simulink model "model"  (R2024b)
settings: Solver=ode1  StartTime=0.0  StopTime=10  FixedStep=0.0001  RelTol=1e-3
values from neighbouring files (symbols this model uses):
  a1 = c*a2    (= 810)    [init.m]
  a2 = c*a3    (= 270)    [init.m]
  a3 = c*a4    (= 90)    [init.m]
  a4 = c*10    (= 30)    [init.m]
  c1 = 50    [init.m]
  c2 = 1    [init.m]
  d = 100    [init.m]
  dis_gain = 30    [init.m]
  epsilon = 1    [init.m]
  i = 20    [init.m]
  k = 5    [init.m]
  mu = 0.9    [init.m]
  p = 400    [init.m]
  phi_frist = 0    [init.m]
  psi_frist = 0    [init.m]
  tau_p_max = 3000000    [init.m]
  theta_frist = 0    [init.m]
  umax = pi/2 - 0.01    (= 1.56079632679)    [init.m]
  w = wo    (= 50)    [init.m]
  wo = 50    [init.m]
  x_frist = 0    [init.m]
  y_frist = 0    [init.m]
  z_frist = 0    [init.m]
libraries: fod x36, slpidlib x6, simulink x1
(part 2 of 4)

== system model/FO_SMC/Subsystem/Subsystem1 ==
  y : Inport
  Constant : Constant  Value=a1
  Constant1 : Constant  Value=a2
  Constant2 : Constant  Value=a3
  Constant3 : Constant  Value=a4
  Demux : Demux
  Integrator : Integrator  InitialCondition=[0]
  MATLAB Function : MATLAB Function  TreatAsAtomicUnit=on
  Mux : Mux
  y_hat : Outport
  y1_hat : Outport  Port=2
  y1_hat1 : Outport  Port=3
  wires:
  Constant3/1 -> MATLAB Function/9(a4)
  Constant2/1 -> MATLAB Function/8(a3)
  Constant1/1 -> MATLAB Function/7(a2)
  Constant/1 -> MATLAB Function/6(a1)
  Demux/4 -> MATLAB Function/5(z4)
  MATLAB Function/4(z4_1) -> Mux/4
  Demux/3 -> MATLAB Function/4(z3), y1_hat1/1
  Integrator/1 -> Demux/1
  MATLAB Function/3(z3_1) -> Mux/3
  Demux/1 -> MATLAB Function/2(z1), y_hat/1
  MATLAB Function/1(z1_1) -> Mux/1
  MATLAB Function/2(z2_1) -> Mux/2
  Mux/1 -> Integrator/1
  Demux/2 -> MATLAB Function/3(z2), y1_hat/1
  y/1 -> MATLAB Function/1(x)

== system model/FO_SMC/Subsystem/Subsystem2 ==
  y : Inport
  Constant : Constant  Value=a1
  Constant1 : Constant  Value=a2
  Constant2 : Constant  Value=a3
  Constant3 : Constant  Value=a4
  Demux : Demux
  Integrator : Integrator  InitialCondition=[0]
  MATLAB Function : MATLAB Function  TreatAsAtomicUnit=on
  Mux : Mux
  y_hat : Outport
  y1_hat : Outport  Port=2
  y1_hat1 : Outport  Port=3
  wires:
  y/1 -> MATLAB Function/1(x)
  Demux/2 -> y1_hat/1, MATLAB Function/3(z2)
  Mux/1 -> Integrator/1
  MATLAB Function/2(z2_1) -> Mux/2
  MATLAB Function/1(z1_1) -> Mux/1
  Demux/1 -> y_hat/1, MATLAB Function/2(z1)
  MATLAB Function/3(z3_1) -> Mux/3
  Integrator/1 -> Demux/1
  Demux/3 -> y1_hat1/1, MATLAB Function/4(z3)
  MATLAB Function/4(z4_1) -> Mux/4
  Demux/4 -> MATLAB Function/5(z4)
  Constant/1 -> MATLAB Function/6(a1)
  Constant1/1 -> MATLAB Function/7(a2)
  Constant2/1 -> MATLAB Function/8(a3)
  Constant3/1 -> MATLAB Function/9(a4)

== system model/FO_SMC/Subsystem/Subsystem3 ==
  y : Inport
  Constant : Constant  Value=a1
  Constant1 : Constant  Value=a2
  Constant2 : Constant  Value=a3
  Constant3 : Constant  Value=a4
  Demux : Demux
  Integrator : Integrator  InitialCondition=[0]
  MATLAB Function : MATLAB Function  TreatAsAtomicUnit=on
  Mux : Mux
  y_hat : Outport
  y1_hat : Outport  Port=2
  y1_hat1 : Outport  Port=3
  wires:
  Constant3/1 -> MATLAB Function/9(a4)
  Constant2/1 -> MATLAB Function/8(a3)
  Constant1/1 -> MATLAB Function/7(a2)
  Constant/1 -> MATLAB Function/6(a1)
  Demux/4 -> MATLAB Function/5(z4)
  MATLAB Function/4(z4_1) -> Mux/4
  Demux/3 -> MATLAB Function/4(z3), y1_hat1/1
  Integrator/1 -> Demux/1
  MATLAB Function/3(z3_1) -> Mux/3
  Demux/1 -> MATLAB Function/2(z1), y_hat/1
  MATLAB Function/1(z1_1) -> Mux/1
  MATLAB Function/2(z2_1) -> Mux/2
  Mux/1 -> Integrator/1
  Demux/2 -> MATLAB Function/3(z2), y1_hat/1
  y/1 -> MATLAB Function/1(x)

== system model/FO_SMC/Subsystem/Subsystem4 ==
  y : Inport
  Constant : Constant  Value=a1
  Constant1 : Constant  Value=a2
  Constant2 : Constant  Value=a3
  Constant3 : Constant  Value=a4
  Demux : Demux
  Integrator : Integrator  InitialCondition=[0]
  MATLAB Function : MATLAB Function  TreatAsAtomicUnit=on
  Mux : Mux
  y_hat : Outport
  y1_hat : Outport  Port=2
  y1_hat1 : Outport  Port=3
  wires:
  y/1 -> MATLAB Function/1(x)
  Demux/2 -> y1_hat/1, MATLAB Function/3(z2)
  Mux/1 -> Integrator/1
  MATLAB Function/2(z2_1) -> Mux/2
  MATLAB Function/1(z1_1) -> Mux/1
  Demux/1 -> y_hat/1, MATLAB Function/2(z1)
  MATLAB Function/3(z3_1) -> Mux/3
  Integrator/1 -> Demux/1
  Demux/3 -> y1_hat1/1, MATLAB Function/4(z3)
  MATLAB Function/4(z4_1) -> Mux/4
  Demux/4 -> MATLAB Function/5(z4)
  Constant/1 -> MATLAB Function/6(a1)
  Constant1/1 -> MATLAB Function/7(a2)
  Constant2/1 -> MATLAB Function/8(a3)
  Constant3/1 -> MATLAB Function/9(a4)

== system model/FO_SMC/Subsystem/Subsystem5 ==
  y : Inport
  Constant : Constant  Value=a1
  Constant1 : Constant  Value=a2
  Constant2 : Constant  Value=a3
  Constant3 : Constant  Value=a4
  Demux : Demux
  Integrator : Integrator  InitialCondition=[0]
  MATLAB Function : MATLAB Function  TreatAsAtomicUnit=on
  Mux : Mux
  y_hat : Outport
  y1_hat : Outport  Port=2
  y1_hat1 : Outport  Port=3
  wires:
  y/1 -> MATLAB Function/1(x)
  Demux/2 -> y1_hat/1, MATLAB Function/3(z2)
  Mux/1 -> Integrator/1
  MATLAB Function/2(z2_1) -> Mux/2
  MATLAB Function/1(z1_1) -> Mux/1
  Demux/1 -> y_hat/1, MATLAB Function/2(z1)
  MATLAB Function/3(z3_1) -> Mux/3
  Integrator/1 -> Demux/1
  Demux/3 -> y1_hat1/1, MATLAB Function/4(z3)
  MATLAB Function/4(z4_1) -> Mux/4
  Demux/4 -> MATLAB Function/5(z4)
  Constant/1 -> MATLAB Function/6(a1)
  Constant1/1 -> MATLAB Function/7(a2)
  Constant2/1 -> MATLAB Function/8(a3)
  Constant3/1 -> MATLAB Function/9(a4)

== system model/FO_SMC/Subsystem/Subsystem6 ==
  y : Inport
  Constant : Constant  Value=a1
  Constant1 : Constant  Value=a2
  Constant2 : Constant  Value=a3
  Constant3 : Constant  Value=a4
  Demux : Demux
  Integrator : Integrator  InitialCondition=[0]
  MATLAB Function : MATLAB Function  TreatAsAtomicUnit=on
  Mux : Mux
  y_hat : Outport
  y1_hat : Outport  Port=2
  y1_hat1 : Outport  Port=3
  wires:
  Constant3/1 -> MATLAB Function/9(a4)
  Constant2/1 -> MATLAB Function/8(a3)
  Constant1/1 -> MATLAB Function/7(a2)
  Constant/1 -> MATLAB Function/6(a1)
  Demux/4 -> MATLAB Function/5(z4)
  MATLAB Function/4(z4_1) -> Mux/4
  Demux/3 -> MATLAB Function/4(z3), y1_hat1/1
  Integrator/1 -> Demux/1
  MATLAB Function/3(z3_1) -> Mux/3
  Demux/1 -> MATLAB Function/2(z1), y_hat/1
  MATLAB Function/1(z1_1) -> Mux/1
  MATLAB Function/2(z2_1) -> Mux/2
  Mux/1 -> Integrator/1
  Demux/2 -> MATLAB Function/3(z2), y1_hat/1
  y/1 -> MATLAB Function/1(x)

== system model/FO_SMC/Subsystem2/Subsystem1 ==
  In1 : Inport
  Demux : Demux  Outputs=6
  Mux : Mux  Inputs=6
  Mux1 : Mux  Inputs=6
  Subsystem1 : Subsystem
  Subsystem2 : Subsystem
  Subsystem3 : Subsystem
  Subsystem4 : Subsystem
  Subsystem5 : Subsystem
  Subsystem6 : Subsystem
  Out1 : Outport
  Out2 : Outport  Port=2
  wires:
  Mux1/1 -> Out2/1
  Subsystem1/2(y1_hat) -> Mux1/2
  Demux/4 -> Subsystem3/1(y)
  Subsystem5/2(y1_hat) -> Mux1/5
  In1/1 -> Demux/1
  Demux/5 -> Subsystem5/1(y)
  Subsystem3/1(y_hat) -> Mux/4
  Subsystem3/2(y1_hat) -> Mux1/4
  Demux/6 -> Subsystem6/1(y)
  Subsystem6/2(y1_hat) -> Mux1/6
  Subsystem4/2(y1_hat) -> Mux1/1
  Subsystem2/1(y_hat) -> Mux/3
  Subsystem1/1(y_hat) -> Mux/2
  Demux/2 -> Subsystem1/1(y)
  Demux/3 -> Subsystem2/1(y)
  Mux/1 -> Out1/1
  Subsystem6/1(y_hat) -> Mux/6
  Demux/1 -> Subsystem4/1(y)
  Subsystem2/2(y1_hat) -> Mux1/3
  Subsystem5/1(y_hat) -> Mux/5
  Subsystem4/1(y_hat) -> Mux/1

== system model/FO_SMC_ESO/LESO/Subsystem1 ==
  eta : Inport
  In2 : Inport  Port=2
  Demux : Demux  Outputs=6
  Demux1 : Demux  Outputs=6
  Mux : Mux  Inputs=6
  Subsystem1 : Subsystem
  Subsystem2 : Subsystem
  Subsystem3 : Subsystem
  Subsystem4 : Subsystem
  Subsystem5 : Subsystem
  Subsystem6 : Subsystem
  tau_1 : Outport
  wires:
  Demux/6 -> Subsystem5/2(tau_0)
  Demux/4 -> Subsystem3/2(tau_0)
  Demux/2 -> Subsystem1/2(tau_0)
  Demux/5 -> Subsystem4/2(tau_0)
  Mux/1 -> tau_1/1
  Demux/3 -> Subsystem2/2(tau_0)
  In2/1 -> Demux/1
  Demux/1 -> Subsystem6/2(tau_0)
  Subsystem6/1(Out3) -> Mux/1
  Subsystem1/1(Out3) -> Mux/2
  Subsystem2/1(Out3) -> Mux/3
  Subsystem3/1(Out3) -> Mux/4
  eta/1 -> Demux1/1
  Demux1/1 -> Subsystem6/1(eta)
  Demux1/2 -> Subsystem1/1(eta)
  Demux1/3 -> Subsystem2/1(eta)
  Demux1/4 -> Subsystem3/1(eta)
  Demux1/5 -> Subsystem4/1(eta)
  Subsystem4/1(Out3) -> Mux/5
  Demux1/6 -> Subsystem5/1(eta)
  Subsystem5/1(Out3) -> Mux/6

== system model/FO_SMC_ESO/Levant微分器/Subsystem1 ==
  y : Inport
  Constant : Constant  Value=a1
  Constant1 : Constant  Value=a2
  Constant2 : Constant  Value=a3
  Constant3 : Constant  Value=a4
  Demux : Demux
  Integrator : Integrator  InitialCondition=[0]
  MATLAB Function : MATLAB Function  TreatAsAtomicUnit=on
  Mux : Mux
  y_hat : Outport
  y1_hat : Outport  Port=2
  y1_hat1 : Outport  Port=3
  wires:
  Constant3/1 -> MATLAB Function/9(a4)
  Constant2/1 -> MATLAB Function/8(a3)
  Constant1/1 -> MATLAB Function/7(a2)
  Constant/1 -> MATLAB Function/6(a1)
  Demux/4 -> MATLAB Function/5(z4)
  MATLAB Function/4(z4_1) -> Mux/4
  Demux/3 -> MATLAB Function/4(z3), y1_hat1/1
  Integrator/1 -> Demux/1
  MATLAB Function/3(z3_1) -> Mux/3
  Demux/1 -> MATLAB Function/2(z1), y_hat/1
  MATLAB Function/1(z1_1) -> Mux/1
  MATLAB Function/2(z2_1) -> Mux/2
  Mux/1 -> Integrator/1
  Demux/2 -> MATLAB Function/3(z2), y1_hat/1
  y/1 -> MATLAB Function/1(x)

== system model/FO_SMC_ESO/Levant微分器/Subsystem2 ==
  y : Inport
  Constant : Constant  Value=a1
  Constant1 : Constant  Value=a2
  Constant2 : Constant  Value=a3
  Constant3 : Constant  Value=a4
  Demux : Demux
  Integrator : Integrator  InitialCondition=[0]
  MATLAB Function : MATLAB Function  TreatAsAtomicUnit=on
  Mux : Mux
  y_hat : Outport
  y1_hat : Outport  Port=2
  y1_hat1 : Outport  Port=3
  wires:
  y/1 -> MATLAB Function/1(x)
  Demux/2 -> y1_hat/1, MATLAB Function/3(z2)
  Mux/1 -> Integrator/1
  MATLAB Function/2(z2_1) -> Mux/2
  MATLAB Function/1(z1_1) -> Mux/1
  Demux/1 -> y_hat/1, MATLAB Function/2(z1)
  MATLAB Function/3(z3_1) -> Mux/3
  Integrator/1 -> Demux/1
  Demux/3 -> y1_hat1/1, MATLAB Function/4(z3)
  MATLAB Function/4(z4_1) -> Mux/4
  Demux/4 -> MATLAB Function/5(z4)
  Constant/1 -> MATLAB Function/6(a1)
  Constant1/1 -> MATLAB Function/7(a2)
  Constant2/1 -> MATLAB Function/8(a3)
  Constant3/1 -> MATLAB Function/9(a4)

== system model/FO_SMC_ESO/Levant微分器/Subsystem3 ==
  y : Inport
  Constant : Constant  Value=a1
  Constant1 : Constant  Value=a2
  Constant2 : Constant  Value=a3
  Constant3 : Constant  Value=a4
  Demux : Demux
  Integrator : Integrator  InitialCondition=[0]
  MATLAB Function : MATLAB Function  TreatAsAtomicUnit=on
  Mux : Mux
  y_hat : Outport
  y1_hat : Outport  Port=2
  y1_hat1 : Outport  Port=3
  wires:
  Constant3/1 -> MATLAB Function/9(a4)
  Constant2/1 -> MATLAB Function/8(a3)
  Constant1/1 -> MATLAB Function/7(a2)
  Constant/1 -> MATLAB Function/6(a1)
  Demux/4 -> MATLAB Function/5(z4)
  MATLAB Function/4(z4_1) -> Mux/4
  Demux/3 -> MATLAB Function/4(z3), y1_hat1/1
  Integrator/1 -> Demux/1
  MATLAB Function/3(z3_1) -> Mux/3
  Demux/1 -> MATLAB Function/2(z1), y_hat/1
  MATLAB Function/1(z1_1) -> Mux/1
  MATLAB Function/2(z2_1) -> Mux/2
  Mux/1 -> Integrator/1
  Demux/2 -> MATLAB Function/3(z2), y1_hat/1
  y/1 -> MATLAB Function/1(x)

== system model/FO_SMC_ESO/Levant微分器/Subsystem4 ==
  y : Inport
  Constant : Constant  Value=a1
  Constant1 : Constant  Value=a2
  Constant2 : Constant  Value=a3
  Constant3 : Constant  Value=a4
  Demux : Demux
  Integrator : Integrator  InitialCondition=[0]
  MATLAB Function : MATLAB Function  TreatAsAtomicUnit=on
  Mux : Mux
  y_hat : Outport
  y1_hat : Outport  Port=2
  y1_hat1 : Outport  Port=3
  wires:
  y/1 -> MATLAB Function/1(x)
  Demux/2 -> y1_hat/1, MATLAB Function/3(z2)
  Mux/1 -> Integrator/1
  MATLAB Function/2(z2_1) -> Mux/2
  MATLAB Function/1(z1_1) -> Mux/1
  Demux/1 -> y_hat/1, MATLAB Function/2(z1)
  MATLAB Function/3(z3_1) -> Mux/3
  Integrator/1 -> Demux/1
  Demux/3 -> y1_hat1/1, MATLAB Function/4(z3)
  MATLAB Function/4(z4_1) -> Mux/4
  Demux/4 -> MATLAB Function/5(z4)
  Constant/1 -> MATLAB Function/6(a1)
  Constant1/1 -> MATLAB Function/7(a2)
  Constant2/1 -> MATLAB Function/8(a3)
  Constant3/1 -> MATLAB Function/9(a4)

== system model/FO_SMC_ESO/Levant微分器/Subsystem5 ==
  y : Inport
  Constant : Constant  Value=a1
  Constant1 : Constant  Value=a2
  Constant2 : Constant  Value=a3
  Constant3 : Constant  Value=a4
  Demux : Demux
  Integrator : Integrator  InitialCondition=[0]
  MATLAB Function : MATLAB Function  TreatAsAtomicUnit=on
  Mux : Mux
  y_hat : Outport
  y1_hat : Outport  Port=2
  y1_hat1 : Outport  Port=3
  wires:
  y/1 -> MATLAB Function/1(x)
  Demux/2 -> y1_hat/1, MATLAB Function/3(z2)
  Mux/1 -> Integrator/1
  MATLAB Function/2(z2_1) -> Mux/2
  MATLAB Function/1(z1_1) -> Mux/1
  Demux/1 -> y_hat/1, MATLAB Function/2(z1)
  MATLAB Function/3(z3_1) -> Mux/3
  Integrator/1 -> Demux/1
  Demux/3 -> y1_hat1/1, MATLAB Function/4(z3)
  MATLAB Function/4(z4_1) -> Mux/4
  Demux/4 -> MATLAB Function/5(z4)
  Constant/1 -> MATLAB Function/6(a1)
  Constant1/1 -> MATLAB Function/7(a2)
  Constant2/1 -> MATLAB Function/8(a3)
  Constant3/1 -> MATLAB Function/9(a4)

== system model/FO_SMC_ESO/Levant微分器/Subsystem6 ==
  y : Inport
  Constant : Constant  Value=a1
  Constant1 : Constant  Value=a2
  Constant2 : Constant  Value=a3
  Constant3 : Constant  Value=a4
  Demux : Demux
  Integrator : Integrator  InitialCondition=[0]
  MATLAB Function : MATLAB Function  TreatAsAtomicUnit=on
  Mux : Mux
  y_hat : Outport
  y1_hat : Outport  Port=2
  y1_hat1 : Outport  Port=3
  wires:
  Constant3/1 -> MATLAB Function/9(a4)
  Constant2/1 -> MATLAB Function/8(a3)
  Constant1/1 -> MATLAB Function/7(a2)
  Constant/1 -> MATLAB Function/6(a1)
  Demux/4 -> MATLAB Function/5(z4)
  MATLAB Function/4(z4_1) -> Mux/4
  Demux/3 -> MATLAB Function/4(z3), y1_hat1/1
  Integrator/1 -> Demux/1
  MATLAB Function/3(z3_1) -> Mux/3
  Demux/1 -> MATLAB Function/2(z1), y_hat/1
  MATLAB Function/1(z1_1) -> Mux/1
  MATLAB Function/2(z2_1) -> Mux/2
  Mux/1 -> Integrator/1
  Demux/2 -> MATLAB Function/3(z2), y1_hat/1
  y/1 -> MATLAB Function/1(x)

== system model/FO_SMC_ESO/Subsystem3/Subsystem2 ==
  eta : Inport
  eta_d : Inport  Port=2
  MATLAB Function6 : MATLAB Function  TreatAsAtomicUnit=on
  Subsystem1 : Subsystem
  D1 : Outport
  D2 : Outport  Port=2
  wires:
  MATLAB Function6/1(e) -> Subsystem1/1(In1)
  eta_d/1 -> MATLAB Function6/2(x_d)
  Subsystem1/1(Out1) -> D1/1
  eta/1 -> MATLAB Function6/1(x)
  Subsystem1/2(Out2) -> D2/1

== system model/FO_SMC_T/Subsystem/Subsystem1 ==
  y : Inport
  Constant : Constant  Value=a1
  Constant1 : Constant  Value=a2
  Constant2 : Constant  Value=a3
  Constant3 : Constant  Value=a4
  Demux : Demux
  Integrator : Integrator  InitialCondition=[0]
  MATLAB Function : MATLAB Function  TreatAsAtomicUnit=on
  Mux : Mux
  y_hat : Outport
  y1_hat : Outport  Port=2
  y1_hat1 : Outport  Port=3
  wires:
  Constant3/1 -> MATLAB Function/9(a4)
  Constant2/1 -> MATLAB Function/8(a3)
  Constant1/1 -> MATLAB Function/7(a2)
  Constant/1 -> MATLAB Function/6(a1)
  Demux/4 -> MATLAB Function/5(z4)
  MATLAB Function/4(z4_1) -> Mux/4
  Demux/3 -> MATLAB Function/4(z3), y1_hat1/1
  Integrator/1 -> Demux/1
  MATLAB Function/3(z3_1) -> Mux/3
  Demux/1 -> MATLAB Function/2(z1), y_hat/1
  MATLAB Function/1(z1_1) -> Mux/1
  MATLAB Function/2(z2_1) -> Mux/2
  Mux/1 -> Integrator/1
  Demux/2 -> MATLAB Function/3(z2), y1_hat/1
  y/1 -> MATLAB Function/1(x)

== system model/FO_SMC_T/Subsystem/Subsystem2 ==
  y : Inport
  Constant : Constant  Value=a1
  Constant1 : Constant  Value=a2
  Constant2 : Constant  Value=a3
  Constant3 : Constant  Value=a4
  Demux : Demux
  Integrator : Integrator  InitialCondition=[0]
  MATLAB Function : MATLAB Function  TreatAsAtomicUnit=on
  Mux : Mux
  y_hat : Outport
  y1_hat : Outport  Port=2
  y1_hat1 : Outport  Port=3
  wires:
  y/1 -> MATLAB Function/1(x)
  Demux/2 -> y1_hat/1, MATLAB Function/3(z2)
  Mux/1 -> Integrator/1
  MATLAB Function/2(z2_1) -> Mux/2
  MATLAB Function/1(z1_1) -> Mux/1
  Demux/1 -> y_hat/1, MATLAB Function/2(z1)
  MATLAB Function/3(z3_1) -> Mux/3
  Integrator/1 -> Demux/1
  Demux/3 -> y1_hat1/1, MATLAB Function/4(z3)
  MATLAB Function/4(z4_1) -> Mux/4
  Demux/4 -> MATLAB Function/5(z4)
  Constant/1 -> MATLAB Function/6(a1)
  Constant1/1 -> MATLAB Function/7(a2)
  Constant2/1 -> MATLAB Function/8(a3)
  Constant3/1 -> MATLAB Function/9(a4)

== system model/FO_SMC_T/Subsystem/Subsystem3 ==
  y : Inport
  Constant : Constant  Value=a1
  Constant1 : Constant  Value=a2
  Constant2 : Constant  Value=a3
  Constant3 : Constant  Value=a4
  Demux : Demux
  Integrator : Integrator  InitialCondition=[0]
  MATLAB Function : MATLAB Function  TreatAsAtomicUnit=on
  Mux : Mux
  y_hat : Outport
  y1_hat : Outport  Port=2
  y1_hat1 : Outport  Port=3
  wires:
  Constant3/1 -> MATLAB Function/9(a4)
  Constant2/1 -> MATLAB Function/8(a3)
  Constant1/1 -> MATLAB Function/7(a2)
  Constant/1 -> MATLAB Function/6(a1)
  Demux/4 -> MATLAB Function/5(z4)
  MATLAB Function/4(z4_1) -> Mux/4
  Demux/3 -> MATLAB Function/4(z3), y1_hat1/1
  Integrator/1 -> Demux/1
  MATLAB Function/3(z3_1) -> Mux/3
  Demux/1 -> MATLAB Function/2(z1), y_hat/1
  MATLAB Function/1(z1_1) -> Mux/1
  MATLAB Function/2(z2_1) -> Mux/2
  Mux/1 -> Integrator/1
  Demux/2 -> MATLAB Function/3(z2), y1_hat/1
  y/1 -> MATLAB Function/1(x)

== system model/FO_SMC_T/Subsystem/Subsystem4 ==
  y : Inport
  Constant : Constant  Value=a1
  Constant1 : Constant  Value=a2
  Constant2 : Constant  Value=a3
  Constant3 : Constant  Value=a4
  Demux : Demux
  Integrator : Integrator  InitialCondition=[0]
  MATLAB Function : MATLAB Function  TreatAsAtomicUnit=on
  Mux : Mux
  y_hat : Outport
  y1_hat : Outport  Port=2
  y1_hat1 : Outport  Port=3
  wires:
  y/1 -> MATLAB Function/1(x)
  Demux/2 -> y1_hat/1, MATLAB Function/3(z2)
  Mux/1 -> Integrator/1
  MATLAB Function/2(z2_1) -> Mux/2
  MATLAB Function/1(z1_1) -> Mux/1
  Demux/1 -> y_hat/1, MATLAB Function/2(z1)
  MATLAB Function/3(z3_1) -> Mux/3
  Integrator/1 -> Demux/1
  Demux/3 -> y1_hat1/1, MATLAB Function/4(z3)
  MATLAB Function/4(z4_1) -> Mux/4
  Demux/4 -> MATLAB Function/5(z4)
  Constant/1 -> MATLAB Function/6(a1)
  Constant1/1 -> MATLAB Function/7(a2)
  Constant2/1 -> MATLAB Function/8(a3)
  Constant3/1 -> MATLAB Function/9(a4)

== system model/FO_SMC_T/Subsystem/Subsystem5 ==
  y : Inport
  Constant : Constant  Value=a1
  Constant1 : Constant  Value=a2
  Constant2 : Constant  Value=a3
  Constant3 : Constant  Value=a4
  Demux : Demux
  Integrator : Integrator  InitialCondition=[0]
  MATLAB Function : MATLAB Function  TreatAsAtomicUnit=on
  Mux : Mux
  y_hat : Outport
  y1_hat : Outport  Port=2
  y1_hat1 : Outport  Port=3
  wires:
  y/1 -> MATLAB Function/1(x)
  Demux/2 -> y1_hat/1, MATLAB Function/3(z2)
  Mux/1 -> Integrator/1
  MATLAB Function/2(z2_1) -> Mux/2
  MATLAB Function/1(z1_1) -> Mux/1
  Demux/1 -> y_hat/1, MATLAB Function/2(z1)
  MATLAB Function/3(z3_1) -> Mux/3
  Integrator/1 -> Demux/1
  Demux/3 -> y1_hat1/1, MATLAB Function/4(z3)
  MATLAB Function/4(z4_1) -> Mux/4
  Demux/4 -> MATLAB Function/5(z4)
  Constant/1 -> MATLAB Function/6(a1)
  Constant1/1 -> MATLAB Function/7(a2)
  Constant2/1 -> MATLAB Function/8(a3)
  Constant3/1 -> MATLAB Function/9(a4)

== system model/FO_SMC_T/Subsystem/Subsystem6 ==
  y : Inport
  Constant : Constant  Value=a1
  Constant1 : Constant  Value=a2
  Constant2 : Constant  Value=a3
  Constant3 : Constant  Value=a4
  Demux : Demux
  Integrator : Integrator  InitialCondition=[0]
  MATLAB Function : MATLAB Function  TreatAsAtomicUnit=on
  Mux : Mux
  y_hat : Outport
  y1_hat : Outport  Port=2
  y1_hat1 : Outport  Port=3
  wires:
  Constant3/1 -> MATLAB Function/9(a4)
  Constant2/1 -> MATLAB Function/8(a3)
  Constant1/1 -> MATLAB Function/7(a2)
  Constant/1 -> MATLAB Function/6(a1)
  Demux/4 -> MATLAB Function/5(z4)
  MATLAB Function/4(z4_1) -> Mux/4
  Demux/3 -> MATLAB Function/4(z3), y1_hat1/1
  Integrator/1 -> Demux/1
  MATLAB Function/3(z3_1) -> Mux/3
  Demux/1 -> MATLAB Function/2(z1), y_hat/1
  MATLAB Function/1(z1_1) -> Mux/1
  MATLAB Function/2(z2_1) -> Mux/2
  Mux/1 -> Integrator/1
  Demux/2 -> MATLAB Function/3(z2), y1_hat/1
  y/1 -> MATLAB Function/1(x)

== system model/FO_SMC_T/Subsystem2/Subsystem1 ==
  In1 : Inport
  Demux : Demux  Outputs=6
  Mux : Mux  Inputs=6
  Mux1 : Mux  Inputs=6
  Subsystem1 : Subsystem
  Subsystem2 : Subsystem
  Subsystem3 : Subsystem
  Subsystem4 : Subsystem
  Subsystem5 : Subsystem
  Subsystem6 : Subsystem
  Out1 : Outport
  Out2 : Outport  Port=2
  wires:
  Mux1/1 -> Out2/1
  Subsystem1/2(y1_hat) -> Mux1/2
  Demux/4 -> Subsystem3/1(y)
  Subsystem5/2(y1_hat) -> Mux1/5
  In1/1 -> Demux/1
  Demux/5 -> Subsystem5/1(y)
  Subsystem3/1(y_hat) -> Mux/4
  Subsystem3/2(y1_hat) -> Mux1/4
  Demux/6 -> Subsystem6/1(y)
  Subsystem6/2(y1_hat) -> Mux1/6
  Subsystem4/2(y1_hat) -> Mux1/1
  Subsystem2/1(y_hat) -> Mux/3
  Subsystem1/1(y_hat) -> Mux/2
  Demux/2 -> Subsystem1/1(y)
  Demux/3 -> Subsystem2/1(y)
  Mux/1 -> Out1/1
  Subsystem6/1(y_hat) -> Mux/6
  Demux/1 -> Subsystem4/1(y)
  Subsystem2/2(y1_hat) -> Mux1/3
  Subsystem5/1(y_hat) -> Mux/5
  Subsystem4/1(y_hat) -> Mux/1

== system model/SMC/Subsystem/Subsystem1 ==
  y : Inport
  Constant : Constant  Value=a1
  Constant1 : Constant  Value=a2
  Constant2 : Constant  Value=a3
  Constant3 : Constant  Value=a4
  Demux : Demux
  Integrator : Integrator  InitialCondition=[0]
  MATLAB Function : MATLAB Function  TreatAsAtomicUnit=on
  Mux : Mux
  y_hat : Outport
  y1_hat : Outport  Port=2
  y1_hat1 : Outport  Port=3
  wires:
  Constant3/1 -> MATLAB Function/9(a4)
  Constant2/1 -> MATLAB Function/8(a3)
  Constant1/1 -> MATLAB Function/7(a2)
  Constant/1 -> MATLAB Function/6(a1)
  Demux/4 -> MATLAB Function/5(z4)
  MATLAB Function/4(z4_1) -> Mux/4
  Demux/3 -> MATLAB Function/4(z3), y1_hat1/1
  Integrator/1 -> Demux/1
  MATLAB Function/3(z3_1) -> Mux/3
  Demux/1 -> MATLAB Function/2(z1), y_hat/1
  MATLAB Function/1(z1_1) -> Mux/1
  MATLAB Function/2(z2_1) -> Mux/2
  Mux/1 -> Integrator/1
  Demux/2 -> MATLAB Function/3(z2), y1_hat/1
  y/1 -> MATLAB Function/1(x)

== system model/SMC/Subsystem/Subsystem2 ==
  y : Inport
  Constant : Constant  Value=a1
  Constant1 : Constant  Value=a2
  Constant2 : Constant  Value=a3
  Constant3 : Constant  Value=a4
  Demux : Demux
  Integrator : Integrator  InitialCondition=[0]
  MATLAB Function : MATLAB Function  TreatAsAtomicUnit=on
  Mux : Mux
  y_hat : Outport
  y1_hat : Outport  Port=2
  y1_hat1 : Outport  Port=3
  wires:
  y/1 -> MATLAB Function/1(x)
  Demux/2 -> y1_hat/1, MATLAB Function/3(z2)
  Mux/1 -> Integrator/1
  MATLAB Function/2(z2_1) -> Mux/2
  MATLAB Function/1(z1_1) -> Mux/1
  Demux/1 -> y_hat/1, MATLAB Function/2(z1)
  MATLAB Function/3(z3_1) -> Mux/3
  Integrator/1 -> Demux/1
  Demux/3 -> y1_hat1/1, MATLAB Function/4(z3)
  MATLAB Function/4(z4_1) -> Mux/4
  Demux/4 -> MATLAB Function/5(z4)
  Constant/1 -> MATLAB Function/6(a1)
  Constant1/1 -> MATLAB Function/7(a2)
  Constant2/1 -> MATLAB Function/8(a3)
  Constant3/1 -> MATLAB Function/9(a4)

== system model/SMC/Subsystem/Subsystem3 ==
  y : Inport
  Constant : Constant  Value=a1
  Constant1 : Constant  Value=a2
  Constant2 : Constant  Value=a3
  Constant3 : Constant  Value=a4
  Demux : Demux
  Integrator : Integrator  InitialCondition=[0]
  MATLAB Function : MATLAB Function  TreatAsAtomicUnit=on
  Mux : Mux
  y_hat : Outport
  y1_hat : Outport  Port=2
  y1_hat1 : Outport  Port=3
  wires:
  Constant3/1 -> MATLAB Function/9(a4)
  Constant2/1 -> MATLAB Function/8(a3)
  Constant1/1 -> MATLAB Function/7(a2)
  Constant/1 -> MATLAB Function/6(a1)
  Demux/4 -> MATLAB Function/5(z4)
  MATLAB Function/4(z4_1) -> Mux/4
  Demux/3 -> MATLAB Function/4(z3), y1_hat1/1
  Integrator/1 -> Demux/1
  MATLAB Function/3(z3_1) -> Mux/3
  Demux/1 -> MATLAB Function/2(z1), y_hat/1
  MATLAB Function/1(z1_1) -> Mux/1
  MATLAB Function/2(z2_1) -> Mux/2
  Mux/1 -> Integrator/1
  Demux/2 -> MATLAB Function/3(z2), y1_hat/1
  y/1 -> MATLAB Function/1(x)

== system model/SMC/Subsystem/Subsystem4 ==
  y : Inport
  Constant : Constant  Value=a1
  Constant1 : Constant  Value=a2
  Constant2 : Constant  Value=a3
  Constant3 : Constant  Value=a4
  Demux : Demux
  Integrator : Integrator  InitialCondition=[0]
  MATLAB Function : MATLAB Function  TreatAsAtomicUnit=on
  Mux : Mux
  y_hat : Outport
  y1_hat : Outport  Port=2
  y1_hat1 : Outport  Port=3
  wires:
  y/1 -> MATLAB Function/1(x)
  Demux/2 -> y1_hat/1, MATLAB Function/3(z2)
  Mux/1 -> Integrator/1
  MATLAB Function/2(z2_1) -> Mux/2
  MATLAB Function/1(z1_1) -> Mux/1
  Demux/1 -> y_hat/1, MATLAB Function/2(z1)
  MATLAB Function/3(z3_1) -> Mux/3
  Integrator/1 -> Demux/1
  Demux/3 -> y1_hat1/1, MATLAB Function/4(z3)
  MATLAB Function/4(z4_1) -> Mux/4
  Demux/4 -> MATLAB Function/5(z4)
  Constant/1 -> MATLAB Function/6(a1)
  Constant1/1 -> MATLAB Function/7(a2)
  Constant2/1 -> MATLAB Function/8(a3)
  Constant3/1 -> MATLAB Function/9(a4)

== system model/SMC/Subsystem/Subsystem5 ==
  y : Inport
  Constant : Constant  Value=a1
  Constant1 : Constant  Value=a2
  Constant2 : Constant  Value=a3
  Constant3 : Constant  Value=a4
  Demux : Demux
  Integrator : Integrator  InitialCondition=[0]
  MATLAB Function : MATLAB Function  TreatAsAtomicUnit=on
  Mux : Mux
  y_hat : Outport
  y1_hat : Outport  Port=2
  y1_hat1 : Outport  Port=3
  wires:
  y/1 -> MATLAB Function/1(x)
  Demux/2 -> y1_hat/1, MATLAB Function/3(z2)
  Mux/1 -> Integrator/1
  MATLAB Function/2(z2_1) -> Mux/2
  MATLAB Function/1(z1_1) -> Mux/1
  Demux/1 -> y_hat/1, MATLAB Function/2(z1)
  MATLAB Function/3(z3_1) -> Mux/3
  Integrator/1 -> Demux/1
  Demux/3 -> y1_hat1/1, MATLAB Function/4(z3)
  MATLAB Function/4(z4_1) -> Mux/4
  Demux/4 -> MATLAB Function/5(z4)
  Constant/1 -> MATLAB Function/6(a1)
  Constant1/1 -> MATLAB Function/7(a2)
  Constant2/1 -> MATLAB Function/8(a3)
  Constant3/1 -> MATLAB Function/9(a4)

== system model/SMC/Subsystem/Subsystem6 ==
  y : Inport
  Constant : Constant  Value=a1
  Constant1 : Constant  Value=a2
  Constant2 : Constant  Value=a3
  Constant3 : Constant  Value=a4
  Demux : Demux
  Integrator : Integrator  InitialCondition=[0]
  MATLAB Function : MATLAB Function  TreatAsAtomicUnit=on
  Mux : Mux
  y_hat : Outport
  y1_hat : Outport  Port=2
  y1_hat1 : Outport  Port=3
  wires:
  Constant3/1 -> MATLAB Function/9(a4)
  Constant2/1 -> MATLAB Function/8(a3)
  Constant1/1 -> MATLAB Function/7(a2)
  Constant/1 -> MATLAB Function/6(a1)
  Demux/4 -> MATLAB Function/5(z4)
  MATLAB Function/4(z4_1) -> Mux/4
  Demux/3 -> MATLAB Function/4(z3), y1_hat1/1
  Integrator/1 -> Demux/1
  MATLAB Function/3(z3_1) -> Mux/3
  Demux/1 -> MATLAB Function/2(z1), y_hat/1
  MATLAB Function/1(z1_1) -> Mux/1
  MATLAB Function/2(z2_1) -> Mux/2
  Mux/1 -> Integrator/1
  Demux/2 -> MATLAB Function/3(z2), y1_hat/1
  y/1 -> MATLAB Function/1(x)

== system model/ADRC/控制器/6路levant微分器/Subsystem1 ==
  y : Inport
  Demux : Demux
  Integrator : Integrator  InitialCondition=[0]
  MATLAB Function : MATLAB Function  TreatAsAtomicUnit=on
  Mux : Mux
  y_hat : Outport
  y1_hat : Outport  Port=2
  y1_hat1 : Outport  Port=3
  wires:
  y/1 -> MATLAB Function/1(x)
  Demux/2 -> y1_hat/1, MATLAB Function/3(z2)
  Mux/1 -> Integrator/1
  MATLAB Function/2(z2_1) -> Mux/2
  MATLAB Function/1(z1_1) -> Mux/1
  Demux/1 -> MATLAB Function/2(z1), y_hat/1
  MATLAB Function/3(z3_1) -> Mux/3
  Integrator/1 -> Demux/1
  Demux/3 -> y1_hat1/1, MATLAB Function/4(z3)
  MATLAB Function/4(z4_1) -> Mux/4
  Demux/4 -> MATLAB Function/5(z4)

== system model/ADRC/控制器/6路levant微分器/Subsystem2 ==
  y : Inport
  Demux : Demux
  Integrator : Integrator  InitialCondition=[0]
  MATLAB Function : MATLAB Function  TreatAsAtomicUnit=on
  Mux : Mux
  y_hat : Outport
  y1_hat : Outport  Port=2
  y1_hat1 : Outport  Port=3
  wires:
  Demux/4 -> MATLAB Function/5(z4)
  MATLAB Function/4(z4_1) -> Mux/4
  Demux/3 -> MATLAB Function/4(z3), y1_hat1/1
  Integrator/1 -> Demux/1
  MATLAB Function/3(z3_1) -> Mux/3
  Demux/1 -> y_hat/1, MATLAB Function/2(z1)
  MATLAB Function/1(z1_1) -> Mux/1
  MATLAB Function/2(z2_1) -> Mux/2
  Mux/1 -> Integrator/1
  Demux/2 -> MATLAB Function/3(z2), y1_hat/1
  y/1 -> MATLAB Function/1(x)

== system model/ADRC/控制器/6路levant微分器/Subsystem3 ==
  y : Inport
  Demux : Demux
  Integrator : Integrator  InitialCondition=[0]
  MATLAB Function : MATLAB Function  TreatAsAtomicUnit=on
  Mux : Mux
  y_hat : Outport
  y1_hat : Outport  Port=2
  y1_hat1 : Outport  Port=3
  wires:
  y/1 -> MATLAB Function/1(x)
  Demux/2 -> y1_hat/1, MATLAB Function/3(z2)
  Mux/1 -> Integrator/1
  MATLAB Function/2(z2_1) -> Mux/2
  MATLAB Function/1(z1_1) -> Mux/1
  Demux/1 -> MATLAB Function/2(z1), y_hat/1
  MATLAB Function/3(z3_1) -> Mux/3
  Integrator/1 -> Demux/1
  Demux/3 -> y1_hat1/1, MATLAB Function/4(z3)
  MATLAB Function/4(z4_1) -> Mux/4
  Demux/4 -> MATLAB Function/5(z4)

== system model/ADRC/控制器/6路levant微分器/Subsystem4 ==
  y : Inport
  Demux : Demux
  Integrator : Integrator  InitialCondition=[0]
  MATLAB Function : MATLAB Function  TreatAsAtomicUnit=on
  Mux : Mux
  y_hat : Outport
  y1_hat : Outport  Port=2
  y1_hat1 : Outport  Port=3
  wires:
  Demux/4 -> MATLAB Function/5(z4)
  MATLAB Function/4(z4_1) -> Mux/4
  Demux/3 -> MATLAB Function/4(z3), y1_hat1/1
  Integrator/1 -> Demux/1
  MATLAB Function/3(z3_1) -> Mux/3
  Demux/1 -> y_hat/1, MATLAB Function/2(z1)
  MATLAB Function/1(z1_1) -> Mux/1
  MATLAB Function/2(z2_1) -> Mux/2
  Mux/1 -> Integrator/1
  Demux/2 -> MATLAB Function/3(z2), y1_hat/1
  y/1 -> MATLAB Function/1(x)

== system model/ADRC/控制器/6路levant微分器/Subsystem5 ==
  y : Inport
  Demux : Demux
  Integrator : Integrator  InitialCondition=[0]
  MATLAB Function : MATLAB Function  TreatAsAtomicUnit=on
  Mux : Mux
  y_hat : Outport
  y1_hat : Outport  Port=2
  y1_hat1 : Outport  Port=3
  wires:
  Demux/4 -> MATLAB Function/5(z4)
  MATLAB Function/4(z4_1) -> Mux/4
  Demux/3 -> MATLAB Function/4(z3), y1_hat1/1
  Integrator/1 -> Demux/1
  MATLAB Function/3(z3_1) -> Mux/3
  Demux/1 -> y_hat/1, MATLAB Function/2(z1)
  MATLAB Function/1(z1_1) -> Mux/1
  MATLAB Function/2(z2_1) -> Mux/2
  Mux/1 -> Integrator/1
  Demux/2 -> MATLAB Function/3(z2), y1_hat/1
  y/1 -> MATLAB Function/1(x)

== system model/ADRC/控制器/6路levant微分器/Subsystem6 ==
  y : Inport
  Demux : Demux
  Integrator : Integrator  InitialCondition=[0]
  MATLAB Function : MATLAB Function  TreatAsAtomicUnit=on
  Mux : Mux
  y_hat : Outport
  y1_hat : Outport  Port=2
  y1_hat1 : Outport  Port=3
  wires:
  y/1 -> MATLAB Function/1(x)
  Demux/2 -> y1_hat/1, MATLAB Function/3(z2)
  Mux/1 -> Integrator/1
  MATLAB Function/2(z2_1) -> Mux/2
  MATLAB Function/1(z1_1) -> Mux/1
  Demux/1 -> MATLAB Function/2(z1), y_hat/1
  MATLAB Function/3(z3_1) -> Mux/3
  Integrator/1 -> Demux/1
  Demux/3 -> y1_hat1/1, MATLAB Function/4(z3)
  MATLAB Function/4(z4_1) -> Mux/4
  Demux/4 -> MATLAB Function/5(z4)

== system model/ADRC/控制器/Subsystem1/Subsystem1 ==
  tau_0 : Inport
  eta : Inport  Port=2
  Constant : Constant  Value=wo
  Demux1 : Demux  Outputs=3
  Integrator : Integrator  InitialCondition=[0;0;0]
  MATLAB Function2 : MATLAB Function  TreatAsAtomicUnit=on
  Out3 : Outport
  Out1 : Outport  Port=2
  Out2 : Outport  Port=3
  wires:
  Demux1/2 -> Out1/1
  Demux1/1 -> Out3/1
  eta/1 -> MATLAB Function2/2(eta)
  MATLAB Function2/1(dh) -> Integrator/1
  Constant/1 -> MATLAB Function2/4(wo)
  Demux1/3 -> Out2/1
  tau_0/1 -> MATLAB Function2/3(tau_0)
  Integrator/1 -> Demux1/1, MATLAB Function2/1(h)

== system model/ADRC/控制器/Subsystem1/Subsystem2 ==
  tau_0 : Inport
  eta : Inport  Port=2
  Constant : Constant  Value=wo
  Demux1 : Demux  Outputs=3
  Integrator : Integrator  InitialCondition=[0;0;0]
  MATLAB Function2 : MATLAB Function  TreatAsAtomicUnit=on
  Out3 : Outport
  Out1 : Outport  Port=2
  Out2 : Outport  Port=3
  wires:
  Integrator/1 -> MATLAB Function2/1(h), Demux1/1
  tau_0/1 -> MATLAB Function2/3(tau_0)
  Demux1/3 -> Out2/1
  Constant/1 -> MATLAB Function2/4(wo)
  MATLAB Function2/1(dh) -> Integrator/1
  eta/1 -> MATLAB Function2/2(eta)
  Demux1/1 -> Out3/1
  Demux1/2 -> Out1/1

== system model/ADRC/控制器/Subsystem1/Subsystem3 ==
  tau_0 : Inport
  eta : Inport  Port=2
  Constant : Constant  Value=wo
  Demux1 : Demux  Outputs=3
  Integrator : Integrator  InitialCondition=[0;0;0]
  MATLAB Function2 : MATLAB Function  TreatAsAtomicUnit=on
  Out3 : Outport
  Out1 : Outport  Port=2
  Out2 : Outport  Port=3
  wires:
  Demux1/2 -> Out1/1
  Demux1/1 -> Out3/1
  eta/1 -> MATLAB Function2/2(eta)
  MATLAB Function2/1(dh) -> Integrator/1
  Constant/1 -> MATLAB Function2/4(wo)
  Demux1/3 -> Out2/1
  tau_0/1 -> MATLAB Function2/3(tau_0)
  Integrator/1 -> Demux1/1, MATLAB Function2/1(h)

== system model/ADRC/控制器/Subsystem1/Subsystem4 ==
  tau_0 : Inport
  eta : Inport  Port=2
  Constant : Constant  Value=wo
  Demux1 : Demux  Outputs=3
  Integrator : Integrator  InitialCondition=[0;0;0]
  MATLAB Function2 : MATLAB Function  TreatAsAtomicUnit=on
  Out3 : Outport
  Out1 : Outport  Port=2
  Out2 : Outport  Port=3
  wires:
  Integrator/1 -> MATLAB Function2/1(h), Demux1/1
  tau_0/1 -> MATLAB Function2/3(tau_0)
  Demux1/3 -> Out2/1
  Constant/1 -> MATLAB Function2/4(wo)
  MATLAB Function2/1(dh) -> Integrator/1
  eta/1 -> MATLAB Function2/2(eta)
  Demux1/1 -> Out3/1
  Demux1/2 -> Out1/1

== system model/ADRC/控制器/Subsystem1/Subsystem5 ==
  tau_0 : Inport
  eta : Inport  Port=2
  Constant : Constant  Value=wo
  Demux1 : Demux  Outputs=3
  Integrator : Integrator  InitialCondition=[0;0;0]
  MATLAB Function2 : MATLAB Function  TreatAsAtomicUnit=on
  Out3 : Outport
  Out1 : Outport  Port=2
  Out2 : Outport  Port=3
  wires:
  Demux1/2 -> Out1/1
  Demux1/1 -> Out3/1
  eta/1 -> MATLAB Function2/2(eta)
  MATLAB Function2/1(dh) -> Integrator/1
  Constant/1 -> MATLAB Function2/4(wo)
  Demux1/3 -> Out2/1
  tau_0/1 -> MATLAB Function2/3(tau_0)
  Integrator/1 -> Demux1/1, MATLAB Function2/1(h)

== system model/ADRC/控制器/Subsystem1/Subsystem6 ==
  tau_0 : Inport
  eta : Inport  Port=2
  Constant : Constant  Value=wo
  Demux1 : Demux  Outputs=3
  Integrator : Integrator  InitialCondition=[0;0;0]
  MATLAB Function2 : MATLAB Function  TreatAsAtomicUnit=on
  Out3 : Outport
  Out1 : Outport  Port=2
  Out2 : Outport  Port=3
  wires:
  Integrator/1 -> MATLAB Function2/1(h), Demux1/1
  tau_0/1 -> MATLAB Function2/3(tau_0)
  Demux1/3 -> Out2/1
  Constant/1 -> MATLAB Function2/4(wo)
  MATLAB Function2/1(dh) -> Integrator/1
  eta/1 -> MATLAB Function2/2(eta)
  Demux1/1 -> Out3/1
  Demux1/2 -> Out1/1

== system model/FO_SMC/Subsystem2/Subsystem1/Subsystem1 ==
  y : Inport
  Fractional operator : fod/Fractional operator  Tag=Fractional operator  K=1  gam=mu-1  ww=[0.001, 1000]  n=5
      settings: SourceProductName=FOMCON Toolbox
  Fractional operator1 : fod/Fractional operator  Tag=Fractional operator  K=1  gam=mu  ww=[0.001, 1000]  n=5
      settings: SourceProductName=FOMCON Toolbox
  y_hat : Outport
  y1_hat : Outport  Port=2
  wires:
  y/1 -> Fractional operator1/1, Fractional operator/1
  Fractional operator/1 -> y_hat/1
  Fractional operator1/1 -> y1_hat/1

== system model/FO_SMC/Subsystem2/Subsystem1/Subsystem2 ==
  y : Inport
  Fractional operator : fod/Fractional operator  Tag=Fractional operator  K=1  gam=mu-1  ww=[0.001, 1000]  n=5
      settings: SourceProductName=FOMCON Toolbox
  Fractional operator1 : fod/Fractional operator  Tag=Fractional operator  K=1  gam=mu  ww=[0.001, 1000]  n=5
      settings: SourceProductName=FOMCON Toolbox
  y_hat : Outport
  y1_hat : Outport  Port=2
  wires:
  Fractional operator1/1 -> y1_hat/1
  Fractional operator/1 -> y_hat/1
  y/1 -> Fractional operator/1, Fractional operator1/1

== system model/FO_SMC/Subsystem2/Subsystem1/Subsystem3 ==
  y : Inport
  Fractional operator : fod/Fractional operator  Tag=Fractional operator  K=1  gam=mu-1  ww=[0.001, 1000]  n=5
      settings: SourceProductName=FOMCON Toolbox
  Fractional operator1 : fod/Fractional operator  Tag=Fractional operator  K=1  gam=mu  ww=[0.001, 1000]  n=5
      settings: SourceProductName=FOMCON Toolbox
  y_hat : Outport
  y1_hat : Outport  Port=2
  wires:
  y/1 -> Fractional operator1/1, Fractional operator/1
  Fractional operator/1 -> y_hat/1
  Fractional operator1/1 -> y1_hat/1

== system model/FO_SMC/Subsystem2/Subsystem1/Subsystem4 ==
  y : Inport
  Fractional operator : fod/Fractional operator  Tag=Fractional operator  K=1  gam=mu-1  ww=[0.001, 1000]  n=5
      settings: SourceProductName=FOMCON Toolbox
  Fractional operator1 : fod/Fractional operator  Tag=Fractional operator  K=1  gam=mu  ww=[0.001, 1000]  n=5
      settings: SourceProductName=FOMCON Toolbox
  y_hat : Outport
  y1_hat : Outport  Port=2
  wires:
  Fractional operator1/1 -> y1_hat/1
  Fractional operator/1 -> y_hat/1
  y/1 -> Fractional operator/1, Fractional operator1/1

== system model/FO_SMC/Subsystem2/Subsystem1/Subsystem5 ==
  y : Inport
  Fractional operator : fod/Fractional operator  Tag=Fractional operator  K=1  gam=mu-1  ww=[0.001, 1000]  n=5
      settings: SourceProductName=FOMCON Toolbox
  Fractional operator1 : fod/Fractional operator  Tag=Fractional operator  K=1  gam=mu  ww=[0.001, 1000]  n=5
      settings: SourceProductName=FOMCON Toolbox
  y_hat : Outport
  y1_hat : Outport  Port=2
  wires:
  Fractional operator1/1 -> y1_hat/1
  Fractional operator/1 -> y_hat/1
  y/1 -> Fractional operator/1, Fractional operator1/1

== system model/FO_SMC/Subsystem2/Subsystem1/Subsystem6 ==
  y : Inport
  Fractional operator : fod/Fractional operator  Tag=Fractional operator  K=1  gam=mu-1  ww=[0.001, 1000]  n=5
      settings: SourceProductName=FOMCON Toolbox
  Fractional operator1 : fod/Fractional operator  Tag=Fractional operator  K=1  gam=mu  ww=[0.001, 1000]  n=5
      settings: SourceProductName=FOMCON Toolbox
  y_hat : Outport
  y1_hat : Outport  Port=2
  wires:
  y/1 -> Fractional operator1/1, Fractional operator/1
  Fractional operator/1 -> y_hat/1
  Fractional operator1/1 -> y1_hat/1

== system model/FO_SMC_ESO/LESO/Subsystem1/Subsystem1 ==
  eta : Inport
  tau_0 : Inport  Port=2
  Constant : Constant  Value=wo
  Demux1 : Demux  Outputs=3
  Integrator : Integrator  InitialCondition=[0;0;0]
  MATLAB Function2 : MATLAB Function  TreatAsAtomicUnit=on
  Out3 : Outport
  wires:
  eta/1 -> MATLAB Function2/2(eta)
  MATLAB Function2/1(dh) -> Integrator/1
  Constant/1 -> MATLAB Function2/4(wo)
  Demux1/3 -> Out3/1
  tau_0/1 -> MATLAB Function2/3(tau_0)
  Integrator/1 -> Demux1/1, MATLAB Function2/1(h)

== system model/FO_SMC_ESO/LESO/Subsystem1/Subsystem2 ==
  eta : Inport
  tau_0 : Inport  Port=2
  Constant : Constant  Value=wo
  Demux1 : Demux  Outputs=3
  Integrator : Integrator  InitialCondition=[0;0;0]
  MATLAB Function2 : MATLAB Function  TreatAsAtomicUnit=on
  Out3 : Outport
  wires:
  Integrator/1 -> MATLAB Function2/1(h), Demux1/1
  tau_0/1 -> MATLAB Function2/3(tau_0)
  Demux1/3 -> Out3/1
  Constant/1 -> MATLAB Function2/4(wo)
  MATLAB Function2/1(dh) -> Integrator/1
  eta/1 -> MATLAB Function2/2(eta)

== system model/FO_SMC_ESO/LESO/Subsystem1/Subsystem3 ==
  eta : Inport
  tau_0 : Inport  Port=2
  Constant : Constant  Value=wo
  Demux1 : Demux  Outputs=3
  Integrator : Integrator  InitialCondition=[0;0;0]
  MATLAB Function2 : MATLAB Function  TreatAsAtomicUnit=on
  Out3 : Outport
  wires:
  eta/1 -> MATLAB Function2/2(eta)
  MATLAB Function2/1(dh) -> Integrator/1
  Constant/1 -> MATLAB Function2/4(wo)
  Demux1/3 -> Out3/1
  tau_0/1 -> MATLAB Function2/3(tau_0)
  Integrator/1 -> Demux1/1, MATLAB Function2/1(h)

== system model/FO_SMC_ESO/LESO/Subsystem1/Subsystem4 ==
  eta : Inport
  tau_0 : Inport  Port=2
  Constant : Constant  Value=wo
  Demux1 : Demux  Outputs=3
  Integrator : Integrator  InitialCondition=[0;0;0]
  MATLAB Function2 : MATLAB Function  TreatAsAtomicUnit=on
  Out3 : Outport
  wires:
  Integrator/1 -> MATLAB Function2/1(h), Demux1/1
  tau_0/1 -> MATLAB Function2/3(tau_0)
  Demux1/3 -> Out3/1
  Constant/1 -> MATLAB Function2/4(wo)
  MATLAB Function2/1(dh) -> Integrator/1
  eta/1 -> MATLAB Function2/2(eta)

== system model/FO_SMC_ESO/LESO/Subsystem1/Subsystem5 ==
  eta : Inport
  tau_0 : Inport  Port=2
  Constant : Constant  Value=wo
  Demux1 : Demux  Outputs=3
  Integrator : Integrator  InitialCondition=[0;0;0]
  MATLAB Function2 : MATLAB Function  TreatAsAtomicUnit=on
  Out3 : Outport
  wires:
  eta/1 -> MATLAB Function2/2(eta)
  MATLAB Function2/1(dh) -> Integrator/1
  Constant/1 -> MATLAB Function2/4(wo)
  Demux1/3 -> Out3/1
  tau_0/1 -> MATLAB Function2/3(tau_0)
  Integrator/1 -> Demux1/1, MATLAB Function2/1(h)

== system model/FO_SMC_ESO/LESO/Subsystem1/Subsystem6 ==
  eta : Inport
  tau_0 : Inport  Port=2
  Constant : Constant  Value=wo
  Demux1 : Demux  Outputs=3
  Integrator : Integrator  InitialCondition=[0;0;0]
  MATLAB Function2 : MATLAB Function  TreatAsAtomicUnit=on
  Out3 : Outport
  wires:
  Integrator/1 -> MATLAB Function2/1(h), Demux1/1
  tau_0/1 -> MATLAB Function2/3(tau_0)
  Demux1/3 -> Out3/1
  Constant/1 -> MATLAB Function2/4(wo)
  MATLAB Function2/1(dh) -> Integrator/1
  eta/1 -> MATLAB Function2/2(eta)

== system model/FO_SMC_ESO/Subsystem3/Subsystem2/Subsystem1 ==
  In1 : Inport
  Demux : Demux  Outputs=6
  Mux : Mux  Inputs=6
  Mux1 : Mux  Inputs=6
  Subsystem1 : Subsystem
  Subsystem2 : Subsystem
  Subsystem3 : Subsystem
  Subsystem4 : Subsystem
  Subsystem5 : Subsystem
  Subsystem6 : Subsystem
  Out1 : Outport
  Out2 : Outport  Port=2
  wires:
  Mux1/1 -> Out2/1
  Subsystem1/2(y1_hat) -> Mux1/2
  Demux/4 -> Subsystem3/1(y)
  Subsystem5/2(y1_hat) -> Mux1/5
  In1/1 -> Demux/1
  Demux/5 -> Subsystem5/1(y)
  Subsystem3/1(y_hat) -> Mux/4
  Subsystem3/2(y1_hat) -> Mux1/4
  Demux/6 -> Subsystem6/1(y)
  Subsystem6/2(y1_hat) -> Mux1/6
  Subsystem4/2(y1_hat) -> Mux1/1
  Subsystem2/1(y_hat) -> Mux/3
  Subsystem1/1(y_hat) -> Mux/2
  Demux/2 -> Subsystem1/1(y)
  Demux/3 -> Subsystem2/1(y)
  Mux/1 -> Out1/1
  Subsystem6/1(y_hat) -> Mux/6
  Demux/1 -> Subsystem4/1(y)
  Subsystem2/2(y1_hat) -> Mux1/3
  Subsystem5/1(y_hat) -> Mux/5
  Subsystem4/1(y_hat) -> Mux/1

== system model/FO_SMC_T/Subsystem2/Subsystem1/Subsystem1 ==
  y : Inport
  Fractional operator : fod/Fractional operator  Tag=Fractional operator  K=1  gam=mu-1  ww=[0.001, 1000]  n=5
      settings: SourceProductName=FOMCON Toolbox
  Fractional operator1 : fod/Fractional operator  Tag=Fractional operator  K=1  gam=mu  ww=[0.001, 1000]  n=5
      settings: SourceProductName=FOMCON Toolbox
  y_hat : Outport
  y1_hat : Outport  Port=2
  wires:
  y/1 -> Fractional operator1/1, Fractional operator/1
  Fractional operator/1 -> y_hat/1
  Fractional operator1/1 -> y1_hat/1

== system model/FO_SMC_T/Subsystem2/Subsystem1/Subsystem2 ==
  y : Inport
  Fractional operator : fod/Fractional operator  Tag=Fractional operator  K=1  gam=mu-1  ww=[0.001, 1000]  n=5
      settings: SourceProductName=FOMCON Toolbox
  Fractional operator1 : fod/Fractional operator  Tag=Fractional operator  K=1  gam=mu  ww=[0.001, 1000]  n=5
      settings: SourceProductName=FOMCON Toolbox
  y_hat : Outport
  y1_hat : Outport  Port=2
  wires:
  Fractional operator1/1 -> y1_hat/1
  Fractional operator/1 -> y_hat/1
  y/1 -> Fractional operator/1, Fractional operator1/1

== system model/FO_SMC_T/Subsystem2/Subsystem1/Subsystem3 ==
  y : Inport
  Fractional operator : fod/Fractional operator  Tag=Fractional operator  K=1  gam=mu-1  ww=[0.001, 1000]  n=5
      settings: SourceProductName=FOMCON Toolbox
  Fractional operator1 : fod/Fractional operator  Tag=Fractional operator  K=1  gam=mu  ww=[0.001, 1000]  n=5
      settings: SourceProductName=FOMCON Toolbox
  y_hat : Outport
  y1_hat : Outport  Port=2
  wires:
  y/1 -> Fractional operator1/1, Fractional operator/1
  Fractional operator/1 -> y_hat/1
  Fractional operator1/1 -> y1_hat/1

== system model/FO_SMC_T/Subsystem2/Subsystem1/Subsystem4 ==
  y : Inport
  Fractional operator : fod/Fractional operator  Tag=Fractional operator  K=1  gam=mu-1  ww=[0.001, 1000]  n=5
      settings: SourceProductName=FOMCON Toolbox
  Fractional operator1 : fod/Fractional operator  Tag=Fractional operator  K=1  gam=mu  ww=[0.001, 1000]  n=5
      settings: SourceProductName=FOMCON Toolbox
  y_hat : Outport
  y1_hat : Outport  Port=2
  wires:
  Fractional operator1/1 -> y1_hat/1
  Fractional operator/1 -> y_hat/1
  y/1 -> Fractional operator/1, Fractional operator1/1

== system model/FO_SMC_T/Subsystem2/Subsystem1/Subsystem5 ==
  y : Inport
  Fractional operator : fod/Fractional operator  Tag=Fractional operator  K=1  gam=mu-1  ww=[0.001, 1000]  n=5
      settings: SourceProductName=FOMCON Toolbox
  Fractional operator1 : fod/Fractional operator  Tag=Fractional operator  K=1  gam=mu  ww=[0.001, 1000]  n=5
      settings: SourceProductName=FOMCON Toolbox
  y_hat : Outport
  y1_hat : Outport  Port=2
  wires:
  Fractional operator1/1 -> y1_hat/1
  Fractional operator/1 -> y_hat/1
  y/1 -> Fractional operator/1, Fractional operator1/1

== system model/FO_SMC_T/Subsystem2/Subsystem1/Subsystem6 ==
  y : Inport
  Fractional operator : fod/Fractional operator  Tag=Fractional operator  K=1  gam=mu-1  ww=[0.001, 1000]  n=5
      settings: SourceProductName=FOMCON Toolbox
  Fractional operator1 : fod/Fractional operator  Tag=Fractional operator  K=1  gam=mu  ww=[0.001, 1000]  n=5
      settings: SourceProductName=FOMCON Toolbox
  y_hat : Outport
  y1_hat : Outport  Port=2
  wires:
  y/1 -> Fractional operator1/1, Fractional operator/1
  Fractional operator/1 -> y_hat/1
  Fractional operator1/1 -> y1_hat/1

== system model/FO_SMC_ESO/Subsystem3/Subsystem2/Subsystem1/Subsystem1 ==
  y : Inport
  Fractional operator : fod/Fractional operator  Tag=Fractional operator  K=1  gam=mu-1  ww=[0.001, 1000]  n=5
      settings: SourceProductName=FOMCON Toolbox
  Fractional operator1 : fod/Fractional operator  Tag=Fractional operator  K=1  gam=mu  ww=[0.001, 1000]  n=5
      settings: SourceProductName=FOMCON Toolbox
  y_hat : Outport
  y1_hat : Outport  Port=2
  wires:
  y/1 -> Fractional operator1/1, Fractional operator/1
  Fractional operator/1 -> y_hat/1
  Fractional operator1/1 -> y1_hat/1

== system model/FO_SMC_ESO/Subsystem3/Subsystem2/Subsystem1/Subsystem2 ==
  y : Inport
  Fractional operator : fod/Fractional operator  Tag=Fractional operator  K=1  gam=mu-1  ww=[0.001, 1000]  n=5
      settings: SourceProductName=FOMCON Toolbox
  Fractional operator1 : fod/Fractional operator  Tag=Fractional operator  K=1  gam=mu  ww=[0.001, 1000]  n=5
      settings: SourceProductName=FOMCON Toolbox
  y_hat : Outport
  y1_hat : Outport  Port=2
  wires:
  Fractional operator1/1 -> y1_hat/1
  Fractional operator/1 -> y_hat/1
  y/1 -> Fractional operator/1, Fractional operator1/1

== system model/FO_SMC_ESO/Subsystem3/Subsystem2/Subsystem1/Subsystem3 ==
  y : Inport
  Fractional operator : fod/Fractional operator  Tag=Fractional operator  K=1  gam=mu-1  ww=[0.001, 1000]  n=5
      settings: SourceProductName=FOMCON Toolbox
  Fractional operator1 : fod/Fractional operator  Tag=Fractional operator  K=1  gam=mu  ww=[0.001, 1000]  n=5
      settings: SourceProductName=FOMCON Toolbox
  y_hat : Outport
  y1_hat : Outport  Port=2
  wires:
  y/1 -> Fractional operator1/1, Fractional operator/1
  Fractional operator/1 -> y_hat/1
  Fractional operator1/1 -> y1_hat/1

== system model/FO_SMC_ESO/Subsystem3/Subsystem2/Subsystem1/Subsystem4 ==
  y : Inport
  Fractional operator : fod/Fractional operator  Tag=Fractional operator  K=1  gam=mu-1  ww=[0.001, 1000]  n=5
      settings: SourceProductName=FOMCON Toolbox
  Fractional operator1 : fod/Fractional operator  Tag=Fractional operator  K=1  gam=mu  ww=[0.001, 1000]  n=5
      settings: SourceProductName=FOMCON Toolbox
  y_hat : Outport
  y1_hat : Outport  Port=2
  wires:
  Fractional operator1/1 -> y1_hat/1
  Fractional operator/1 -> y_hat/1
  y/1 -> Fractional operator/1, Fractional operator1/1

== system model/FO_SMC_ESO/Subsystem3/Subsystem2/Subsystem1/Subsystem5 ==
  y : Inport
  Fractional operator : fod/Fractional operator  Tag=Fractional operator  K=1  gam=mu-1  ww=[0.001, 1000]  n=5
      settings: SourceProductName=FOMCON Toolbox
  Fractional operator1 : fod/Fractional operator  Tag=Fractional operator  K=1  gam=mu  ww=[0.001, 1000]  n=5
      settings: SourceProductName=FOMCON Toolbox
  y_hat : Outport
  y1_hat : Outport  Port=2
  wires:
  Fractional operator1/1 -> y1_hat/1
  Fractional operator/1 -> y_hat/1
  y/1 -> Fractional operator/1, Fractional operator1/1

== system model/FO_SMC_ESO/Subsystem3/Subsystem2/Subsystem1/Subsystem6 ==
  y : Inport
  Fractional operator : fod/Fractional operator  Tag=Fractional operator  K=1  gam=mu-1  ww=[0.001, 1000]  n=5
      settings: SourceProductName=FOMCON Toolbox
  Fractional operator1 : fod/Fractional operator  Tag=Fractional operator  K=1  gam=mu  ww=[0.001, 1000]  n=5
      settings: SourceProductName=FOMCON Toolbox
  y_hat : Outport
  y1_hat : Outport  Port=2
  wires:
  y/1 -> Fractional operator1/1, Fractional operator/1
  Fractional operator/1 -> y_hat/1
  Fractional operator1/1 -> y1_hat/1

== matlab function model/eta_d_sin/MATLAB Function1 ==
  data: t input; y output
function y = fcn(t)
    
y = [15*cos(5*t);20*cos(5*t);25*cos(5*t)];

== matlab function model/eta_d_sin/MATLAB Function2 ==
  data: t input; y output
function y = fcn(t)
    
y = [-75*sin(5*t);-100*sin(5*t);-125*sin(5*t)];

== matlab function model/eta_d_y/MATLAB Function ==
  data: t input; y output
function y = fcn(t)
    
y = [3*sin(0.04*pi*t);3*cos(0.04*pi*t);0.3*t];

== matlab function model/FO_SMC_ESO/Subsystem3/Subsystem2/MATLAB Function6 ==
  data: x input; e output size=6; x_d input
function e  = fcn(x,x_d)

e = x - x_d;
